simulink model "VDSE_2018a"  (R2018a)
settings: Solver=ode5  StartTime=0.0  StopTime=T_simulation  FixedStep=simulation_step_time  RelTol=1e-3
values from neighbouring files (symbols this model uses):
  A = 2    [vehicle_parameters_script.m]
  bump_height = 0    [vehicle_parameters_script.m]
  bump_length = 1    [vehicle_parameters_script.m]
  bump_time = 1    [vehicle_parameters_script.m]
  Bxf = 17.156    [BCD_Parameters.m]
  Bxr = 17.156    [BCD_Parameters.m]
  Byf = 12.71    [BCD_Parameters.m]
  Byr = 12.71    [BCD_Parameters.m]
  cd = 0.35    [vehicle_parameters_script.m]
  central_diff = 1    [vehicle_parameters_script.m]
  cF = 5000    [vehicle_parameters_script.m]
  clF = -0.15    [vehicle_parameters_script.m]
  clR = -0.20    (= -0.2)    [vehicle_parameters_script.m]
  cp_FA = 30    [vehicle_parameters_script.m]
  cp_RA = 13    [vehicle_parameters_script.m]
  cR = 5000    [vehicle_parameters_script.m]
  ctF = tireF.VERTICAL_DAMPING    [vehicle_parameters_script.m]
  ctR = tireR.VERTICAL_DAMPING    [vehicle_parameters_script.m]
  Cxf = 1.406    [BCD_Parameters.m]
  Cxr = 1.406    [BCD_Parameters.m]
  Cyf = 1.63    [BCD_Parameters.m]
  Cyr = 1.63    [BCD_Parameters.m]
  Dxf = 1.2    [BCD_Parameters.m]
  Dxr = 1.2    [BCD_Parameters.m]
  Dyf = 1.1    [BCD_Parameters.m]
  Dyr = 1.8    [BCD_Parameters.m]
  enableDriverControl = 0    [vehicle_parameters_script.m]
  enableLongDynamics = 1    [vehicle_parameters_script.m]
  enablePowertrain = 1    [vehicle_parameters_script.m]
  front_dr = 3.8    [vehicle_parameters_script.m]
  g = 9.806    [vehicle_parameters_script.m]
  Gear_numbers = [1 2 3 4 5 6]    [vehicle_parameters_script.m]
  GR = [2.9 1.8 1.3 1 0.85 0.75]    [vehicle_parameters_script.m]
  hcog = 0.5    [vehicle_parameters_script.m]
  hpc = 0.0    (= 0)    [vehicle_parameters_script.m]
  hrcF = 0.3    [vehicle_parameters_script.m]
  hrcg = (hrcF*lR+hrcR*lF)/(lF+lR)    (= 0.25108)    [vehicle_parameters_script.m]
  hrcR = 0.2    [vehicle_parameters_script.m]
  huFcog = 0.32    [vehicle_parameters_script.m]
  huRcog = 0.32    [vehicle_parameters_script.m]
  initial_gear = 1    [vehicle_parameters_script.m]
  JwF = 2.45    [vehicle_parameters_script.m]
  JwR = 2.45    [vehicle_parameters_script.m]
  Jx = 430    [vehicle_parameters_script.m]
  Jy = 1309    [vehicle_parameters_script.m]
  Jz = 1461    [vehicle_parameters_script.m]
  kF = 40000    [vehicle_parameters_script.m]
  kR = 35000    [vehicle_parameters_script.m]
  kRF = 0    [vehicle_parameters_script.m]
  kRR = 0    [vehicle_parameters_script.m]
  ktF = tireF.VERTICAL_STIFFNESS    [vehicle_parameters_script.m]
  ktR = tireR.VERTICAL_STIFFNESS    [vehicle_parameters_script.m]
  lF = 1.223    [vehicle_parameters_script.m]
  lR = l-lF    (= 1.277)    [vehicle_parameters_script.m]
  m = 1310    [vehicle_parameters_script.m]
  max_pressure = 1000    [vehicle_parameters_script.m]
  maxrpm = 4000    [vehicle_parameters_script.m]
  mF = 45    [vehicle_parameters_script.m]
  minrpm = 1500    [vehicle_parameters_script.m]
  mR = 50    [vehicle_parameters_script.m]
  output_samping_time = 0.001    [vehicle_parameters_script.m]
  phi0 = 0    [vehicle_parameters_script.m]
  phi_dot0 = 0    [vehicle_parameters_script.m]
  psi0 = 0    [vehicle_parameters_script.m]
  psi_dot0 = 0    [vehicle_parameters_script.m]
  rear_dr = 3.8    [vehicle_parameters_script.m]
  requested_speed = 100/3.6    (= 27.7777777778)    [vehicle_parameters_script.m]
  rF = tireF.UNLOADED_RADIUS    [vehicle_parameters_script.m]
  rho = 1.2    [vehicle_parameters_script.m]
  RPMME = Engine(:,1)    [vehicle_parameters_script.m]
  rR = tireR.UNLOADED_RADIUS    [vehicle_parameters_script.m]
  steer_ratio = 13.25    [vehicle_parameters_script.m]
  TFL = 0    [vehicle_parameters_script.m]
  TFR = 0    [vehicle_parameters_script.m]
  theta0 = 0    [vehicle_parameters_script.m]
  theta_dot0 = 0    [vehicle_parameters_script.m]
  TorqueME = []    [vehicle_parameters_script.m]
  TRL = 0    [vehicle_parameters_script.m]
  TRR = 0    [vehicle_parameters_script.m]
  Vx0 = 100/3.6    (= 27.7777777778)    [vehicle_parameters_script.m]
  Vy0 = 0    [vehicle_parameters_script.m]
  Vz0 = 0    [vehicle_parameters_script.m]
  wF = 1.578    [vehicle_parameters_script.m]
  wR = 1.544    [vehicle_parameters_script.m]
  x0 = 0    [vehicle_parameters_script.m]
  xcog_overall = (2*mR*xR+2*xF*mF+m*xs)/(m+2*mF+2*mR)    (= 1.23475333333)    [vehicle_parameters_script.m]
  y0 = 0    [vehicle_parameters_script.m]
  z0 = 0    [vehicle_parameters_script.m]
  zFL0 = 0    [vehicle_parameters_script.m]
  zFL_dot0 = 0    [vehicle_parameters_script.m]
  zFR0 = 0    [vehicle_parameters_script.m]
  zFR_dot0 = 0    [vehicle_parameters_script.m]
  zRL0 = 0    [vehicle_parameters_script.m]
  zRL_dot0 = 0    [vehicle_parameters_script.m]
  zRR0 = 0    [vehicle_parameters_script.m]
  zRR_dot0 = 0    [vehicle_parameters_script.m]
undefined symbols (not defined in the file or in its folder): exf, exr, eyf, eyr, FNOMINf, FNOMINr, PCX1f, PCX1r, PCY1f, PCY1r, PDX1f, PDX1r, PDX2f, PDX2r, PDY1f, PDY1r, PDY2f, PDY2r, PDY3f, PDY3r, PEX1f, PEX1r, PEX2f, PEX2r, PEX3f, PEX3r, PEX4f, PEX4r, PEY1f, PEY1r, PEY2f, PEY2r, PEY3f, PEY3r, PEY4f, PEY4r, PHX1f, PHX1r, PHX2f, PHX2r, PHY1f, PHY1r, PHY2f, PHY2r, PHY3f, PHY3r, PKX1f, PKX1r, PKX2f, PKX2r, PKX3f, PKX3r, PKY1f, PKY1r, PKY2f, PKY2r, PKY3f, PKY3r, PVX1f, PVX1r ... (+122)
libraries: simulink x7, mfeval_LIB x4
(part 3 of 6)

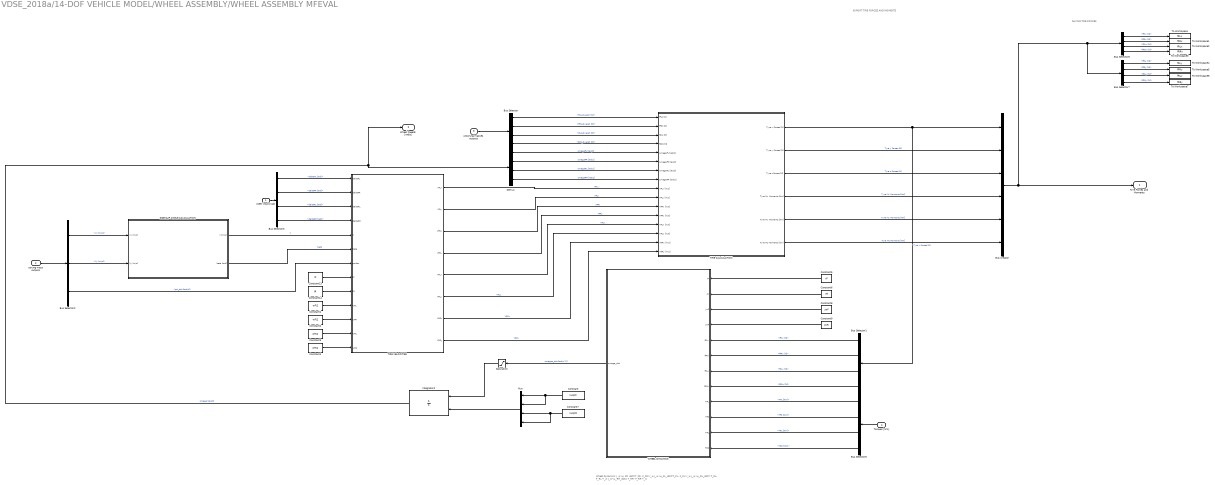
== system VDSE_2018a/14-DOF VEHICLE MODEL/WHEEL ASSEMBLY/WHEEL ASSEMBLY MFEVAL ==
  note: EXPORT TIRE FORCES AND MOMENTS
  note: Wheel Dynamics:
      |
      | J_w∙ω_FR_dot=T_FR- F_FR∙r_w
      | J_w∙ω_FL_dot=T_FL- F_FL∙r_w
      | J_w∙ω_RL_dot= T_RL- F_RL∙r_w
      | J_w∙ω_RR_dot= T_RR- F_RR∙r_w
  note: SAVING TIRE FORCES
  steer input [rad] : Inport
  sprung mass outputs : Inport  Port=2
  unsprung masses outputs : Inport  Port=3
  Torques [Nm] : Inport  Port=4
  Bus Creator : BusCreator  Inputs=6
  Bus Selector : BusSelector  OutputSignals=Unsprung masses z Forces [N].FLz_Overall [N],Unsprung masses z Forces [N].FRz_Overall [N],Unsprung masses z Forces [N].RLz_Overall [N],Unsprung masses z Forces [N].RRz_Overall [N]
  Bus Selector1 : BusSelector  OutputSignals=fFLx [N],fFRx [N],fRLx [N],fRRx [N]
  Bus Selector2 : BusSelector  OutputSignals=Longitudinal Dynamics.Vx [m/s],Lateral Dynamics.Vy [m/s],Yaw dynamics.psi_dot [rad/s]
  Bus Selector3 : BusSelector  OutputSignals=Steering.deltaFL [rad],Steering.deltaFR [rad],Steering.deltaRL [rad],Steering.deltaRR [rad]
  Bus Selector5 : BusSelector  OutputSignals=TFL [Nm],TFR [Nm],TRL [Nm],TRR [Nm]
  Bus Selector6 : BusSelector  OutputSignals=Tyre x Forces [N].fFLx [N],Tyre x Forces [N].fFRx [N],Tyre x Forces [N].fRLx [N],Tyre x Forces [N].fRRx [N]
  Bus Selector7 : BusSelector  OutputSignals=Tyre y Forces [N].fFLy [N],Tyre y Forces [N].fFRy [N],Tyre y Forces [N].fRLy [N],Tyre y Forces [N].fRRy [N]
  Constant : Constant  Value=Vx0/rF
  Constant1 : Constant  Value=wF/2
  Constant13 : Constant  Value=lF
  Constant14 : Constant  Value=lR
  Constant2 : Constant  Value=wF/2
  Constant3 : Constant  Value=wR/2
  Constant4 : Constant  Value=wR/2
  Constant5 : Constant  Value=rF
  Constant6 : Constant  Value=rR
  Constant7 : Constant  Value=Vx0/rR
  Constant8 : Constant  Value=JwF
  Constant9 : Constant  Value=JwR
  Demux : Demux
  Integrator2 : Integrator  InitialConditionSource=external
  Mux : Mux
  SIDE SLIP ANGLE CALCULATION : Subsystem
  Saturation : Saturate  UpperLimit=5000  LowerLimit=-5000
  TIRE CALCULATION : Subsystem
  TIRE VELOCITIES : MATLAB Function  TreatAsAtomicUnit=on
  To Workspace : ToWorkspace  VariableName=fFLx  SaveFormat=Timeseries  SampleTime=-1
  To Workspace1 : ToWorkspace  VariableName=fFRx  SaveFormat=Timeseries  SampleTime=-1
  To Workspace2 : ToWorkspace  VariableName=fRLx  SaveFormat=Timeseries  SampleTime=-1
  To Workspace3 : ToWorkspace  VariableName=fRRx  SaveFormat=Timeseries  SampleTime=-1
  To Workspace4 : ToWorkspace  VariableName=fFLy  SaveFormat=Timeseries  SampleTime=-1
  To Workspace5 : ToWorkspace  VariableName=fFRy  SaveFormat=Timeseries  SampleTime=-1
  To Workspace6 : ToWorkspace  VariableName=fRLy  SaveFormat=Timeseries  SampleTime=-1
  To Workspace7 : ToWorkspace  VariableName=fRRy  SaveFormat=Timeseries  SampleTime=-1
  WHEEL DYNAMICS : MATLAB Function  TreatAsAtomicUnit=on
  Tyre Forces and Moments : Outport
  Wheel Speeds [rad/s] : Outport  Port=2
  wires:
  TIRE CALCULATION/4(Tyre Mx Moments [Nm]) -> Bus Creator/4  "Tyre Mx Moments [Nm]"
  Bus Selector7/4 -> To Workspace7/1  "<fRRy [N]>"
  Bus Selector7/3 -> To Workspace6/1  "<fRLy [N]>"
  Bus Selector7/2 -> To Workspace5/1  "<fFRy [N]>"
  Bus Selector7/1 -> To Workspace4/1  "<fFLy [N]>"
  Bus Selector6/4 -> To Workspace3/1  "<fRRx [N]>"
  Bus Selector6/3 -> To Workspace2/1  "<fRLx [N]>"
  Bus Selector6/2 -> To Workspace1/1  "<fFRx [N]>"
  Bus Selector6/1 -> To Workspace/1  "<fFLx [N]>"
  Torques [Nm]/1 -> Bus Selector5/1
  Bus Creator/1 -> Bus Selector6/1, Bus Selector7/1, Tyre Forces and Moments/1
  steer input [rad]/1 -> Bus Selector3/1
  Bus Selector3/3 -> TIRE VELOCITIES/3(deltaRL)  "<deltaRL [rad]>"
  Bus Selector3/1 -> TIRE VELOCITIES/1(deltaFL)  "<deltaFL [rad]>"
  Bus Selector3/4 -> TIRE VELOCITIES/4(deltaRR)  "<deltaRR [rad]>"
  Bus Selector3/2 -> TIRE VELOCITIES/2(deltaFR)  "<deltaFR [rad]>"
  sprung mass outputs/1 -> Bus Selector2/1
  Bus Selector2/3 -> TIRE VELOCITIES/7(psidot)  "<psi_dot [rad/s]>"
  unsprung masses outputs/1 -> Bus Selector/1
  Bus Selector/2 -> TIRE CALCULATION/2(fFRz [N])  "<FRz_Overall [N]>"
  Bus Selector/3 -> TIRE CALCULATION/3(fRLz [N])  "<RLz_Overall [N]>"
  Bus Selector/4 -> TIRE CALCULATION/4(fRRz [N])  "<RRz_Overall [N]>"
  Bus Selector/1 -> TIRE CALCULATION/1(fFLz [N])  "<FLz_Overall [N]>"
  SIDE SLIP ANGLE CALCULATION/1(V [m/s]) -> TIRE VELOCITIES/5(V)  "V"
  SIDE SLIP ANGLE CALCULATION/2(beta [rad]) -> TIRE VELOCITIES/6(beta)  "beta"
  TIRE VELOCITIES/8(VRRy) -> TIRE CALCULATION/16(VRRy [m/s])  "VRRy"
  TIRE VELOCITIES/7(VRRx) -> TIRE CALCULATION/15(VRRx [m/s])  "VRRx"
  TIRE VELOCITIES/6(VRLy) -> TIRE CALCULATION/14(VRLy [m/s])  "VRLy"
  TIRE VELOCITIES/3(VFRx) -> TIRE CALCULATION/11(VFRx [m/s])  "VFRx"
  Bus Selector1/1 -> WHEEL DYNAMICS/5(fFLx)  "<fFLx [N]>"
  Constant9/1 -> WHEEL DYNAMICS/4(JwR)
  Constant3/1 -> TIRE VELOCITIES/12(wRL)
  TIRE VELOCITIES/5(VRLx) -> TIRE CALCULATION/13(VRLx [m/s])  "VRLx"
  Constant2/1 -> TIRE VELOCITIES/11(wFR)
  Demux/4 -> TIRE CALCULATION/8(omegaRR [rad/s])  "omegaRR [rad/s]"
  Constant/1 -> Mux/1, Mux/2
  Demux/3 -> TIRE CALCULATION/7(omegaRL [rad/s])  "omegaRL [rad/s]"
  Demux/1 -> TIRE CALCULATION/5(omegaFL [rad/s])  "omegaFL [rad/s]"
  WHEEL DYNAMICS/1(omega_dot) -> Saturation/1  "omegas_dot [rad/s^2]"
  Constant14/1 -> TIRE VELOCITIES/9(lR)
  Constant8/1 -> WHEEL DYNAMICS/3(JwF)
  Constant1/1 -> TIRE VELOCITIES/10(wFL)
  Mux/1 -> Integrator2/2
  Constant5/1 -> WHEEL DYNAMICS/1(rF)
  Constant13/1 -> TIRE VELOCITIES/8(lF)
  Integrator2/1 -> Wheel Speeds [rad/s]/1, Demux/1  "omega [rad/s]"
  Bus Selector1/2 -> WHEEL DYNAMICS/6(fFRx)  "<fFRx [N]>"
  Constant4/1 -> TIRE VELOCITIES/13(wRR)
  Bus Selector1/3 -> WHEEL DYNAMICS/7(fRLx)  "<fRLx [N]>"
  TIRE VELOCITIES/4(VFRy) -> TIRE CALCULATION/12(VFRy [m/s])  "VFRy"
  TIRE VELOCITIES/1(VFLx) -> TIRE CALCULATION/9(VFLx [m/s])  "VFLx"
  Constant6/1 -> WHEEL DYNAMICS/2(rR)
  Demux/2 -> TIRE CALCULATION/6(omegaFR [rad/s])  "omegaFR [rad/s]"
  Constant7/1 -> Mux/4, Mux/3
  Bus Selector1/4 -> WHEEL DYNAMICS/8(fRRx)  "<fRRx [N]>"
  TIRE VELOCITIES/2(VFLy) -> TIRE CALCULATION/10(VFLy [m/s])  "VFLy"
  TIRE CALCULATION/1(Tyre x Forces [N]) -> Bus Creator/1, Bus Selector1/1  "Tyre x Forces [N]"
  TIRE CALCULATION/2(Tyre y Forces [N]) -> Bus Creator/2  "Tyre y Forces [N]"
  TIRE CALCULATION/6(Tyre Mz Moments [Nm]) -> Bus Creator/6  "Tyre Mz Moments [Nm]"
  TIRE CALCULATION/3(Tyre z Forces [N]) -> Bus Creator/3  "Tyre z Forces [N]"
  TIRE CALCULATION/5(Tyre My Moments [Nm]) -> Bus Creator/5  "Tyre My Moments [Nm]"
  Bus Selector2/2 -> SIDE SLIP ANGLE CALCULATION/2(Vy [m/s])  "<Vy [m/s]>"
  Bus Selector2/1 -> SIDE SLIP ANGLE CALCULATION/1(Vx [m/s])  "<Vx [m/s]>"
  Bus Selector5/1 -> WHEEL DYNAMICS/9(TFL)  "<TFL [Nm]>"
  Bus Selector5/2 -> WHEEL DYNAMICS/10(TFR)  "<TFR [Nm]>"
  Bus Selector5/3 -> WHEEL DYNAMICS/11(TRL)  "<TRL [Nm]>"
  Bus Selector5/4 -> WHEEL DYNAMICS/12(TRR)  "<TRR [Nm]>"
  Saturation/1 -> Integrator2/1

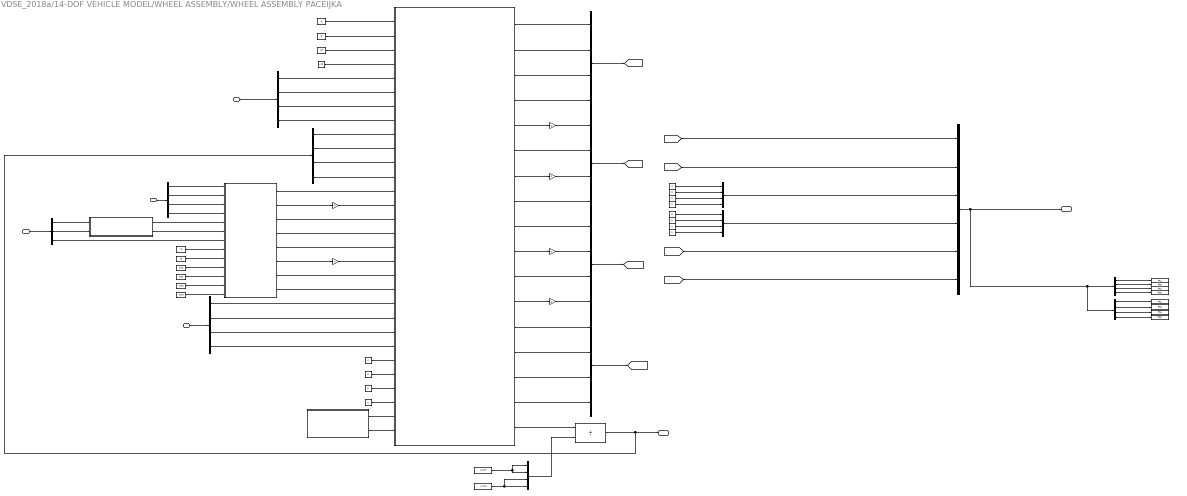
== system VDSE_2018a/14-DOF VEHICLE MODEL/WHEEL ASSEMBLY/WHEEL ASSEMBLY PACEIJKA ==
  note: EXPORTING TIRE FORCES AND MOMENTS
  note: SAVING TIRE FORCES
  steer input [rad] : Inport
  sprung mass outputs : Inport  Port=2
  unsprung masses outputs : Inport  Port=3
  Torques [Nm] : Inport  Port=4
  Bus Creator : BusCreator  Inputs=6
  Bus Creator{1..4,7..8} (6 alike) : BusCreator  Inputs=4
  Bus Selector : BusSelector  OutputSignals=Unsprung masses z Forces [N].FLz_Overall [N],Unsprung masses z Forces [N].FRz_Overall [N],Unsprung masses z Forces [N].RLz_Overall [N],Unsprung masses z Forces [N].RRz_Overall [N]
  Bus Selector2 : BusSelector  OutputSignals=Longitudinal Dynamics.Vx [m/s],Lateral Dynamics.Vy [m/s],Yaw dynamics.psi_dot [rad/s]
  Bus Selector3 : BusSelector  OutputSignals=Steering.deltaFL [rad],Steering.deltaFR [rad],Steering.deltaRL [rad],Steering.deltaRR [rad]
  Bus Selector5 : BusSelector  OutputSignals=TFL [Nm],TFR [Nm],TRL [Nm],TRR [Nm]
  Bus Selector6 : BusSelector  OutputSignals=Tyre x Forces [N].fFLx [N],Tyre x Forces [N].fFRx [N],Tyre x Forces [N].fRLx [N],Tyre x Forces [N].fRRx [N]
  Bus Selector7 : BusSelector  OutputSignals=Tyre y Forces [N].fFLy [N],Tyre y Forces [N].fFRy [N],Tyre y Forces [N].fRLy [N],Tyre y Forces [N].fRRy [N]
  Constant{,26..28} (4 alike) : Constant  Value=0
  Constant1 : Constant  Value=wF/2
  Constant13 : Constant  Value=lF
  Constant14 : Constant  Value=lR
  Constant2 : Constant  Value=wF/2
  Constant20 : Constant  Value=rF
  Constant21 : Constant  Value=rR
  Constant22 : Constant  Value=JwF
  Constant23 : Constant  Value=JwR
  Constant24 : Constant  Value=Vx0/rF
  Constant25 : Constant  Value=Vx0/rR
  Constant3 : Constant  Value=wR/2
  Constant4 : Constant  Value=wR/2
  Demux1 : Demux
  Gain{,1..5} (6 alike) : Gain  Gain=-1
  Integrator1 : Integrator  InitialConditionSource=external
  Mux2 : Mux
  SIDE SLIP ANGLE CALCULATION : Subsystem
  TIRE FORCES AND WHEEL DYNAMICS : MATLAB Function  TreatAsAtomicUnit=on
  TIRE PARAMETERS : Subsystem
  TIRE VELOCITIES : MATLAB Function  TreatAsAtomicUnit=on
  To Workspace : ToWorkspace  VariableName=fFLx  SaveFormat=Timeseries  SampleTime=-1
  To Workspace1 : ToWorkspace  VariableName=fFRx  SaveFormat=Timeseries  SampleTime=-1
  To Workspace2 : ToWorkspace  VariableName=fRLx  SaveFormat=Timeseries  SampleTime=-1
  To Workspace3 : ToWorkspace  VariableName=fRRx  SaveFormat=Timeseries  SampleTime=-1
  To Workspace4 : ToWorkspace  VariableName=fFLy  SaveFormat=Timeseries  SampleTime=-1
  To Workspace5 : ToWorkspace  VariableName=fFRy  SaveFormat=Timeseries  SampleTime=-1
  To Workspace6 : ToWorkspace  VariableName=fRLy  SaveFormat=Timeseries  SampleTime=-1
  To Workspace7 : ToWorkspace  VariableName=fRRy  SaveFormat=Timeseries  SampleTime=-1
  Zero{,1..7} (8 alike) : Constant  Value=0  OutDataTypeStr=Inherit: Inherit via back propagation
  Tyre Forces and Moments : Outport
  Wheel Speeds [rad/s] : Outport  Port=2
  wires:
  Zero/1 -> Bus Creator3/1  "fFLz [N]"
  Zero2/1 -> Bus Creator3/3  "fRLz [N]"
  Zero4/1 -> Bus Creator4/1  "mFLx [Nm]"
  Zero1/1 -> Bus Creator3/2  "fFRz [N]"
  Zero7/1 -> Bus Creator4/4  "mRRx [Nm]"
  Zero5/1 -> Bus Creator4/2  "mFRx [Nm]"
  Zero3/1 -> Bus Creator3/4  "fRRz [N]"
  Zero6/1 -> Bus Creator4/3  "mRLx [Nm]"
  Bus Creator2/1 -> [Tyre_y_Forces]  "Tyre y Forces [N]"
  TIRE FORCES AND WHEEL DYNAMICS/7(fRLy) -> Gain2/1  "fRLy [N]"
  TIRE FORCES AND WHEEL DYNAMICS/5(fFLy) -> Gain3/1  "fFLy [N]"
  Bus Creator1/1 -> [Tyre_x_Forces]  "Tyre x Forces [N]"
  TIRE VELOCITIES/8(VRRy) -> TIRE FORCES AND WHEEL DYNAMICS/20(VRRy)  "VRRy"
  TIRE VELOCITIES/7(VRRx) -> TIRE FORCES AND WHEEL DYNAMICS/19(VRRx)  "VRRx"
  Integrator1/1 -> Wheel Speeds [rad/s]/1, Demux1/1  "omega [rad/s]"
  Demux1/4 -> TIRE FORCES AND WHEEL DYNAMICS/12(omegaRR)
  Demux1/3 -> TIRE FORCES AND WHEEL DYNAMICS/11(omegaRL)
  Demux1/2 -> TIRE FORCES AND WHEEL DYNAMICS/10(omegaFR)
  Demux1/1 -> TIRE FORCES AND WHEEL DYNAMICS/9(omegaFL)
  TIRE FORCES AND WHEEL DYNAMICS/17(omega_dot) -> Integrator1/1  "omegas_dot [rad/s^2]"
  Constant25/1 -> Mux2/4, Mux2/3
  Mux2/1 -> Integrator1/2
  Constant24/1 -> Mux2/1, Mux2/2
  Constant21/1 -> TIRE FORCES AND WHEEL DYNAMICS/2(rR)
  Constant23/1 -> TIRE FORCES AND WHEEL DYNAMICS/4(JwR)
  Constant22/1 -> TIRE FORCES AND WHEEL DYNAMICS/3(JwF)
  Constant20/1 -> TIRE FORCES AND WHEEL DYNAMICS/1(rF)
  TIRE VELOCITIES/2(VFLy) -> Gain/1  "VFLy"
  TIRE VELOCITIES/1(VFLx) -> TIRE FORCES AND WHEEL DYNAMICS/13(VFLx)  "VFLx"
  TIRE VELOCITIES/4(VFRy) -> TIRE FORCES AND WHEEL DYNAMICS/16(VFRy)  "VFRy"
  Constant4/1 -> TIRE VELOCITIES/13(wRR)
  Constant13/1 -> TIRE VELOCITIES/8(lF)
  Constant1/1 -> TIRE VELOCITIES/10(wFL)
  Constant14/1 -> TIRE VELOCITIES/9(lR)
  Constant2/1 -> TIRE VELOCITIES/11(wFR)
  TIRE VELOCITIES/5(VRLx) -> TIRE FORCES AND WHEEL DYNAMICS/17(VRLx)  "VRLx"
  Constant3/1 -> TIRE VELOCITIES/12(wRL)
  TIRE VELOCITIES/3(VFRx) -> TIRE FORCES AND WHEEL DYNAMICS/15(VFRx)  "VFRx"
  TIRE VELOCITIES/6(VRLy) -> Gain1/1  "VRLy"
  SIDE SLIP ANGLE CALCULATION/2(beta [rad]) -> TIRE VELOCITIES/6(beta)  "beta"
  SIDE SLIP ANGLE CALCULATION/1(V [m/s]) -> TIRE VELOCITIES/5(V)  "V"
  Bus Selector/1 -> TIRE FORCES AND WHEEL DYNAMICS/5(fFLz)  "<FLz_Overall [N]>"
  Bus Selector/4 -> TIRE FORCES AND WHEEL DYNAMICS/8(fRRz)  "<RRz_Overall [N]>"
  Bus Selector/3 -> TIRE FORCES AND WHEEL DYNAMICS/7(fRLz)  "<RLz_Overall [N]>"
  Bus Selector/2 -> TIRE FORCES AND WHEEL DYNAMICS/6(fFRz)  "<FRz_Overall [N]>"
  unsprung masses outputs/1 -> Bus Selector/1
  sprung mass outputs/1 -> Bus Selector2/1
  Bus Selector3/2 -> TIRE VELOCITIES/2(deltaFR)  "<deltaFR [rad]>"
  Bus Selector3/4 -> TIRE VELOCITIES/4(deltaRR)  "<deltaRR [rad]>"
  Bus Selector3/1 -> TIRE VELOCITIES/1(deltaFL)  "<deltaFL [rad]>"
  Bus Selector3/3 -> TIRE VELOCITIES/3(deltaRL)  "<deltaRL [rad]>"
  steer input [rad]/1 -> Bus Selector3/1
  Bus Creator/1 -> Bus Selector7/1, Bus Selector6/1, Tyre Forces and Moments/1
  Torques [Nm]/1 -> Bus Selector5/1
  Bus Selector6/1 -> To Workspace/1  "<fFLx [N]>"
  Bus Selector6/2 -> To Workspace1/1  "<fFRx [N]>"
  Bus Selector6/3 -> To Workspace2/1  "<fRLx [N]>"
  Bus Selector6/4 -> To Workspace3/1  "<fRRx [N]>"
  Bus Selector7/1 -> To Workspace4/1  "<fFLy [N]>"
  Bus Selector7/2 -> To Workspace5/1  "<fFRy [N]>"
  Bus Selector7/3 -> To Workspace6/1  "<fRLy [N]>"
  Bus Selector7/4 -> To Workspace7/1  "<fRRy [N]>"
  [Tyre_y_Moments] -> Bus Creator/5  "Tyre My Moments [Nm]"
  Constant/1 -> TIRE FORCES AND WHEEL DYNAMICS/25(gammaFL)
  Constant26/1 -> TIRE FORCES AND WHEEL DYNAMICS/26(gammaFR)
  Constant27/1 -> TIRE FORCES AND WHEEL DYNAMICS/27(gammaRL)
  Constant28/1 -> TIRE FORCES AND WHEEL DYNAMICS/28(gammaRR)
  TIRE PARAMETERS/1(Tire Parameters Front Axle) -> TIRE FORCES AND WHEEL DYNAMICS/29(TireParams_front)
  TIRE PARAMETERS/2(Tire Parameters Rear Axle) -> TIRE FORCES AND WHEEL DYNAMICS/30(TireParams_rear)
  Gain/1 -> TIRE FORCES AND WHEEL DYNAMICS/14(VFLy)  "VFLy"
  Gain1/1 -> TIRE FORCES AND WHEEL DYNAMICS/18(VRLy)  "VRLy"
  TIRE FORCES AND WHEEL DYNAMICS/1(fFLx) -> Bus Creator1/1  "fFLx [N]"
  TIRE FORCES AND WHEEL DYNAMICS/2(fFRx) -> Bus Creator1/2  "fFRx [N]"
  TIRE FORCES AND WHEEL DYNAMICS/3(fRLx) -> Bus Creator1/3  "fRLx [N]"
  TIRE FORCES AND WHEEL DYNAMICS/4(fRRx) -> Bus Creator1/4  "fRRx [N]"
  Gain3/1 -> Bus Creator2/1  "fFLy [N]"
  TIRE FORCES AND WHEEL DYNAMICS/6(fFRy) -> Bus Creator2/2  "fFRy [N]"
  Gain2/1 -> Bus Creator2/3  "fRLy [N]"
  TIRE FORCES AND WHEEL DYNAMICS/8(fRRy) -> Bus Creator2/4  "fRRy [N]"
  [Tyre_x_Forces] -> Bus Creator/1  "Tyre x Forces [N]"
  [Tyre_y_Forces] -> Bus Creator/2  "Tyre y Forces [N]"
  Bus Creator3/1 -> Bus Creator/3  "Tyre z Forces [N]"
  Bus Creator4/1 -> Bus Creator/4  "Tyre Mx Moments [Nm]"
  [Tyre_z_Moments] -> Bus Creator/6  "Tyre Mz Moments [Nm]"
  TIRE FORCES AND WHEEL DYNAMICS/9(mFLz) -> Bus Creator7/1  "mFLz [Nm]"
  TIRE FORCES AND WHEEL DYNAMICS/10(mFRz) -> Gain4/1  "mFRz [Nm]"
  Gain4/1 -> Bus Creator7/2  "mFRz [Nm]"
  TIRE FORCES AND WHEEL DYNAMICS/11(mRLz) -> Bus Creator7/3  "mRLz [Nm]"
  TIRE FORCES AND WHEEL DYNAMICS/12(mRRz) -> Gain5/1  "mRRz [Nm]"
  Gain5/1 -> Bus Creator7/4  "mRRz [Nm]"
  TIRE FORCES AND WHEEL DYNAMICS/13(mFLy) -> Bus Creator8/1  "mFLy [Nm]"
  TIRE FORCES AND WHEEL DYNAMICS/14(mFRy) -> Bus Creator8/2  "mFRy [Nm]"
  TIRE FORCES AND WHEEL DYNAMICS/15(mRLy) -> Bus Creator8/3  "mRLy [Nm]"
  TIRE FORCES AND WHEEL DYNAMICS/16(mRRy) -> Bus Creator8/4  "mRRy [Nm]"
  Bus Creator7/1 -> [Tyre_z_Moments]  "Tyre Mz Moments [Nm]"
  Bus Creator8/1 -> [Tyre_y_Moments]  "Tyre My Moments [Nm]"
  Bus Selector2/1 -> SIDE SLIP ANGLE CALCULATION/1(Vx [m/s])  "<Vx [m/s]>"
  Bus Selector2/2 -> SIDE SLIP ANGLE CALCULATION/2(Vy [m/s])  "<Vy [m/s]>"
  Bus Selector2/3 -> TIRE VELOCITIES/7(psidot)  "<psi_dot [rad/s]>"
  Bus Selector5/1 -> TIRE FORCES AND WHEEL DYNAMICS/21(TFL)  "<TFL [Nm]>"
  Bus Selector5/2 -> TIRE FORCES AND WHEEL DYNAMICS/22(TFR)  "<TFR [Nm]>"
  Bus Selector5/3 -> TIRE FORCES AND WHEEL DYNAMICS/23(TRL)  "<TRL [Nm]>"
  Bus Selector5/4 -> TIRE FORCES AND WHEEL DYNAMICS/24(TRR)  "<TRR [Nm]>"

== system VDSE_2018a/14-DOF VEHICLE MODEL/EQUATIONS OF MOTION FOR CHASSIS/Pitch Dynamics/Downforce ==
  Vx : Inport
  Gain : Gain  Gain=-0.5*rho*clF*A
  Gain{1,3,5,7} (4 alike) : Gain  Gain=0.5
  Gain2 : Gain  Gain=-0.5*rho*clF*A
  Gain4 : Gain  Gain=-0.5*rho*clR*A
  Gain6 : Gain  Gain=-0.5*rho*clR*A
  Square{,1..3} (4 alike) : Math  Operator=square  SaturateOnIntegerOverflow=on
  fFLz_overall : Outport
  fFRz_overall : Outport  Port=2
  fRLz_overall : Outport  Port=3
  fRRz_overall : Outport  Port=4
  wires:
  Gain/1 -> Gain1/1
  Square/1 -> Gain/1
  Gain1/1 -> fFLz_overall/1
  Square1/1 -> Gain2/1
  Gain2/1 -> Gain3/1
  Gain3/1 -> fFRz_overall/1
  Vx/1 -> Square/1, Square1/1, Square2/1, Square3/1
  Gain6/1 -> Gain7/1
  Square3/1 -> Gain6/1
  Square2/1 -> Gain4/1
  Gain4/1 -> Gain5/1
  Gain5/1 -> fRLz_overall/1
  Gain7/1 -> fRRz_overall/1

== system VDSE_2018a/14-DOF VEHICLE MODEL/EQUATIONS OF MOTION FOR CHASSIS/Roll Dynamics/Downforce ==
  Vx : Inport
  Gain : Gain  Gain=-0.5*rho*clF*A
  Gain{1,3,5,7} (4 alike) : Gain  Gain=0.5
  Gain2 : Gain  Gain=-0.5*rho*clF*A
  Gain4 : Gain  Gain=-0.5*rho*clR*A
  Gain6 : Gain  Gain=-0.5*rho*clR*A
  Square{,1..3} (4 alike) : Math  Operator=square  SaturateOnIntegerOverflow=on
  fFLz_overall : Outport
  fFRz_overall : Outport  Port=2
  fRLz_overall : Outport  Port=3
  fRRz_overall : Outport  Port=4
  wires:
  Gain/1 -> Gain1/1
  Square/1 -> Gain/1
  Gain1/1 -> fFLz_overall/1
  Square1/1 -> Gain2/1
  Gain2/1 -> Gain3/1
  Gain3/1 -> fFRz_overall/1
  Vx/1 -> Square/1, Square1/1, Square2/1, Square3/1
  Gain6/1 -> Gain7/1
  Square3/1 -> Gain6/1
  Square2/1 -> Gain4/1
  Gain4/1 -> Gain5/1
  Gain5/1 -> fRLz_overall/1
  Gain7/1 -> fRRz_overall/1

== system VDSE_2018a/14-DOF VEHICLE MODEL/EQUATIONS OF MOTION FOR CHASSIS/Vertical Dynamics/Downforce ==
  Vx : Inport
  Gain : Gain  Gain=-0.5*rho*clF*A
  Gain{1,3,5,7} (4 alike) : Gain  Gain=0.5
  Gain2 : Gain  Gain=-0.5*rho*clF*A
  Gain4 : Gain  Gain=-0.5*rho*clR*A
  Gain6 : Gain  Gain=-0.5*rho*clR*A
  Square{,1..3} (4 alike) : Math  Operator=square  SaturateOnIntegerOverflow=on
  fFLz_overall : Outport
  fFRz_overall : Outport  Port=2
  fRLz_overall : Outport  Port=3
  fRRz_overall : Outport  Port=4
  wires:
  Gain/1 -> Gain1/1
  Square/1 -> Gain/1
  Gain1/1 -> fFLz_overall/1
  Square1/1 -> Gain2/1
  Gain2/1 -> Gain3/1
  Gain3/1 -> fFRz_overall/1
  Vx/1 -> Square/1, Square1/1, Square2/1, Square3/1
  Gain6/1 -> Gain7/1
  Square3/1 -> Gain6/1
  Square2/1 -> Gain4/1
  Gain4/1 -> Gain5/1
  Gain5/1 -> fRLz_overall/1
  Gain7/1 -> fRRz_overall/1

== system VDSE_2018a/14-DOF VEHICLE MODEL/POWERTRAIN AND BRAKES/Engine and Gear Box/Subsystem ==
  Gear_Ratio : Inport
  Front shaft rotational velocity [rpm] : Inport  Port=2
  Rear shaft rotational velocity [rpm] : Inport  Port=3
  Add : Sum
  Gain15 : Gain  Gain=1-central_diff
  Gain16 : Gain  Gain=central_diff
  Product2 : Product
  Product3 : Product
  Engine shaft rotational velocity [rpm] : Outport
  wires:
  Front shaft rotational velocity [rpm]/1 -> Product2/2
  Gear_Ratio/1 -> Product3/1, Product2/1
  Product3/1 -> Gain15/1  "rpm"
  Product2/1 -> Gain16/1
  Gain15/1 -> Add/2
  Rear shaft rotational velocity [rpm]/1 -> Product3/2
  Gain16/1 -> Add/1
  Add/1 -> Engine shaft rotational velocity [rpm]/1

== system VDSE_2018a/14-DOF VEHICLE MODEL/POWERTRAIN AND BRAKES/Engine and Gear Box/Subsystem1 ==
  Engine rpm : Inport
  1-D Lookup Table : Lookup_n-D  NumberOfTableDimensions=1  BreakpointsForDimension1=Gear_numbers  Table=GR  ExtrapMethod=Clip  InternalRulePriority=Speed  RndMeth=Simplest  InputSameDT=on
  Constant : Constant  Value=initial_gear
  Constant1 : Constant  Value=enableDriverControl
  Constant2 : Constant  Value=minrpm
  Constant3 : Constant  Value=maxrpm
  Delay : Delay  DelayLength=1  InitialCondition=initial_gear
  Delay1 : Delay  DelayLength=1  InitialCondition=800
  MATLAB Function : MATLAB Function  TreatAsAtomicUnit=on
  Switch : Switch  Criteria=u2 > Threshold
  Gear No. : Outport
  Gear_Ratio : Outport  Port=2
  wires:
  Delay1/1 -> MATLAB Function/1(rpm)
  Constant2/1 -> MATLAB Function/3(minrpm)
  Delay/1 -> MATLAB Function/2(gr_no_previous)
  Constant1/1 -> Switch/2
  1-D Lookup Table/1 -> Gear_Ratio/1  "Gear_Ratio"
  MATLAB Function/1(gr_no) -> Gear No./1, Switch/1, Delay/1  "Gear No."
  Constant/1 -> Switch/3
  Switch/1 -> 1-D Lookup Table/1
  Constant3/1 -> MATLAB Function/4(maxrpm)
  Engine rpm/1 -> Delay1/1

== system VDSE_2018a/14-DOF VEHICLE MODEL/SUSPENSION/FRONT SUSPENSION/SUSPENSION FL ==
  z [m] : Inport
  Vz [m/s] : Inport  Port=2
  phi [rad] : Inport  Port=3
  phi_dot [rad/s] : Inport  Port=4
  theta [rad] : Inport  Port=5
  theta_dot [rad/s] : Inport  Port=6
  zFR [m] : Inport  Port=7
  yFL_road [m] : Inport  Port=8
  FL : Subsystem
  TIRE VERTICAL DEFLECTION : Subsystem
  fFLz [N] : Outport
  zFL_dot [m/s] : Outport  Port=2
  zFL [m] : Outport  Port=3
  wires:
  FL/2(zFL_dot [m/s]) -> TIRE VERTICAL DEFLECTION/2(zFL_dot [m/s]), zFL_dot [m/s]/1
  z [m]/1 -> FL/1(z [m])
  TIRE VERTICAL DEFLECTION/1(fFLz [N]) -> fFLz [N]/1
  theta [rad]/1 -> FL/5(theta [rad])
  zFR [m]/1 -> FL/7(zFR [m])
  Vz [m/s]/1 -> FL/2(Vz [m/s])
  yFL_road [m]/1 -> TIRE VERTICAL DEFLECTION/3(yFL_road [m]), FL/8(yFL_road [m])
  phi_dot [rad/s]/1 -> FL/4(phi_dot [rad/s])
  FL/1(zFL [m]) -> TIRE VERTICAL DEFLECTION/1(zFL [m]), zFL [m]/1
  phi [rad]/1 -> FL/3(phi [rad])
  theta_dot [rad/s]/1 -> FL/6(theta_dot [rad/s])

== system VDSE_2018a/14-DOF VEHICLE MODEL/SUSPENSION/FRONT SUSPENSION/SUSPENSION FR ==
  z [m] : Inport
  Vz [m/s] : Inport  Port=2
  phi [rad] : Inport  Port=3
  phi_dot [rad/s] : Inport  Port=4
  theta [rad] : Inport  Port=5
  theta_dot [rad/s] : Inport  Port=6
  zFL [m] : Inport  Port=7
  yFR_road [m] : Inport  Port=8
  FR : Subsystem
  TIRE VERTICAL DEFLECTION : Subsystem
  fFRz [N] : Outport
  zFR [m] : Outport  Port=2
  zFR_dot [m/s] : Outport  Port=3
  wires:
  FR/2(zFR_dot [m/s]) -> zFR_dot [m/s]/1, TIRE VERTICAL DEFLECTION/2(zFR_dot [m/s])
  yFR_road [m]/1 -> FR/8(yFR_road [m]), TIRE VERTICAL DEFLECTION/3(yFR_road [m])
  z [m]/1 -> FR/1(z [m])
  TIRE VERTICAL DEFLECTION/1(fFRz [N]) -> fFRz [N]/1
  theta [rad]/1 -> FR/5(theta [rad])
  zFL [m]/1 -> FR/7(zFL [m])
  Vz [m/s]/1 -> FR/2(Vz [m/s])
  phi_dot [rad/s]/1 -> FR/4(phi_dot [rad/s])
  FR/1(zFR [m]) -> TIRE VERTICAL DEFLECTION/1(zFR [m]), zFR [m]/1
  phi [rad]/1 -> FR/3(phi [rad])
  theta_dot [rad/s]/1 -> FR/6(theta_dot [rad/s])

== system VDSE_2018a/14-DOF VEHICLE MODEL/SUSPENSION/Load Transfer/Coupling of load transfer and suspension reaction ==
  Longidutinal Load Transfer [N] : Inport
  Lateral Load Transfer - Front [N] : Inport  Port=2
  Lateral Load Transfer - Rear [N] : Inport  Port=3
  <fFLz [N]> : Inport  Port=4
  <fFRz [N]> : Inport  Port=5
  <fRLz [N]> : Inport  Port=6
  <fRRz [N]> : Inport  Port=7
  Add{,1..4} (5 alike) : Sum
  Add5 : Sum  Inputs=+-
  Add6 : Sum  Inputs=-+
  Add7 : Sum  Inputs=--
  Lateral Load Transfer - Front [N]1 : InportShadow  Port=2
  Lateral Load Transfer - Rear [N]1 : InportShadow  Port=3
  Longidutinal Load Transfer [N]1 : InportShadow
  Longidutinal Load Transfer [N]2 : InportShadow
  Longidutinal Load Transfer [N]3 : InportShadow
  FLz_Overall [N] : Outport
  FRz_Overall [N] : Outport  Port=2
  RLz_Overall [N] : Outport  Port=3
  RRz_Overall [N] : Outport  Port=4
  wires:
  <fFRz [N]>/1 -> Add1/2
  Lateral Load Transfer - Rear [N]/1 -> Add5/2
  Longidutinal Load Transfer [N]/1 -> Add7/1
  Add7/1 -> Add/1  "FL Dynamic LT"
  Lateral Load Transfer - Front [N]/1 -> Add7/2
  Add4/1 -> Add3/1  "RR Dynamic LT"
  Add6/1 -> Add1/1  "FR Dynamic LT"
  Add5/1 -> Add2/1  "RL Dynamic LT"
  <fRRz [N]>/1 -> Add3/2
  <fFLz [N]>/1 -> Add/2
  <fRLz [N]>/1 -> Add2/2
  Add1/1 -> FRz_Overall [N]/1  "FRz_Overall [N]"
  Add3/1 -> RRz_Overall [N]/1  "RRz_Overall [N]"
  Add/1 -> FLz_Overall [N]/1  "FLz_Overall [N]"
  Add2/1 -> RLz_Overall [N]/1  "RLz_Overall [N]"
  Longidutinal Load Transfer [N]1/1 -> Add6/1
  Longidutinal Load Transfer [N]2/1 -> Add5/1
  Longidutinal Load Transfer [N]3/1 -> Add4/1
  Lateral Load Transfer - Front [N]1/1 -> Add6/2
  Lateral Load Transfer - Rear [N]1/1 -> Add4/2

== system VDSE_2018a/14-DOF VEHICLE MODEL/SUSPENSION/Load Transfer/Dynamic Lateral Load Transfer - Front ==
  ay [m/s^2] : Inport
  Add : Sum
  Gain : Gain  Gain=lR/(lR+lF)
  Gain1 : Gain  Gain=2*mF*huFcog/wF
  Gain2 : Gain  Gain=m*hrcF/wF
  Lat. Dynamic Transfer [N] : Outport
  wires:
  ay [m/s^2]/1 -> Gain2/1, Gain1/1
  Gain2/1 -> Gain/1
  Add/1 -> Lat. Dynamic Transfer [N]/1
  Gain1/1 -> Add/2
  Gain/1 -> Add/1

== system VDSE_2018a/14-DOF VEHICLE MODEL/SUSPENSION/Load Transfer/Dynamic Lateral Load Transfer - Rear ==
  ay [m/s^2] : Inport
  Add : Sum
  Gain : Gain  Gain=lF/(lR+lF)
  Gain1 : Gain  Gain=2*mR*huRcog/wR
  Gain2 : Gain  Gain=m*hrcR/wR
  Lat. Dynamic Transfer [N] : Outport
  wires:
  Add/1 -> Lat. Dynamic Transfer [N]/1
  Gain1/1 -> Add/2
  ay [m/s^2]/1 -> Gain2/1, Gain1/1
  Gain2/1 -> Gain/1
  Gain/1 -> Add/1

== system VDSE_2018a/14-DOF VEHICLE MODEL/SUSPENSION/Load Transfer/Dynamic Longitudinal Load Transfer ==
  ax [m/s^2] : Inport
  Add : Sum
  Gain : Gain  Gain=1/2*hpc*m/(lF+lR)/2
  Gain1 : Gain  Gain=(mF*huFcog + mR*huRcog)/(lF+lR)
  Long. Dynamic Transfer [N] : Outport
  wires:
  ax [m/s^2]/1 -> Gain1/1, Gain/1
  Gain/1 -> Add/1
  Add/1 -> Long. Dynamic Transfer [N]/1
  Gain1/1 -> Add/2

== system VDSE_2018a/14-DOF VEHICLE MODEL/SUSPENSION/REAR SUSPENSION/SUSPENSION RL ==
  z [m] : Inport
  Vz [m/s] : Inport  Port=2
  phi [rad] : Inport  Port=3
  phi_dot [rad/s] : Inport  Port=4
  theta [rad] : Inport  Port=5
  theta_dot [rad/s] : Inport  Port=6
  zRR [m] : Inport  Port=7
  yRL_road [m] : Inport  Port=8
  RL : Subsystem
  TIRE VERTICAL DEFLECTION : Subsystem
  fRLz [N] : Outport
  zRL_dot [m/s] : Outport  Port=2
  zRL [m] : Outport  Port=3
  wires:
  RL/2(zRL_dot [m/s]) -> TIRE VERTICAL DEFLECTION/2(zRL_dot [m/s]), zRL_dot [m/s]/1
  z [m]/1 -> RL/1(z [m])
  TIRE VERTICAL DEFLECTION/1(fRLz [N]) -> fRLz [N]/1  "fRLz [N]"
  theta [rad]/1 -> RL/5(theta [rad])
  zRR [m]/1 -> RL/7(zRR [m])
  Vz [m/s]/1 -> RL/2(Vz [m/s])
  yRL_road [m]/1 -> TIRE VERTICAL DEFLECTION/3(yRL_road [m]), RL/8(yRL_road [m])
  phi_dot [rad/s]/1 -> RL/4(phi_dot [rad/s])
  RL/1(zRL [m]) -> TIRE VERTICAL DEFLECTION/1(zRL [m]), zRL [m]/1
  phi [rad]/1 -> RL/3(phi [rad])
  theta_dot [rad/s]/1 -> RL/6(theta_dot [rad/s])

== system VDSE_2018a/14-DOF VEHICLE MODEL/SUSPENSION/REAR SUSPENSION/SUSPENSION RR ==
  z [m] : Inport
  Vz [m/s] : Inport  Port=2
  phi [rad] : Inport  Port=3
  phi_dot [rad/s] : Inport  Port=4
  theta [rad] : Inport  Port=5
  theta_dot [rad/s] : Inport  Port=6
  zRL [m] : Inport  Port=7
  yRR_road [m] : Inport  Port=8
  RR : Subsystem
  TIRE VERTICAL DEFLECTION : Subsystem
  fRRz [N] : Outport
  zRR [m] : Outport  Port=2
  zRR_dot [m/s] : Outport  Port=3
  wires:
  RR/2(zRR_dot [m/s]) -> TIRE VERTICAL DEFLECTION/2(zRR_dot [m/s]), zRR_dot [m/s]/1
  yRR_road [m]/1 -> TIRE VERTICAL DEFLECTION/3(yRR_road [m]), RR/8(yRR_road [m])
  z [m]/1 -> RR/1(z [m])
  TIRE VERTICAL DEFLECTION/1(fRRz [N]) -> fRRz [N]/1
  theta [rad]/1 -> RR/5(theta [rad])
  zRL [m]/1 -> RR/7(zRL [m])
  Vz [m/s]/1 -> RR/2(Vz [m/s])
  phi_dot [rad/s]/1 -> RR/4(phi_dot [rad/s])
  RR/1(zRR [m]) -> TIRE VERTICAL DEFLECTION/1(zRR [m]), zRR [m]/1
  phi [rad]/1 -> RR/3(phi [rad])
  theta_dot [rad/s]/1 -> RR/6(theta_dot [rad/s])

== system VDSE_2018a/14-DOF VEHICLE MODEL/WHEEL ASSEMBLY/WHEEL ASSEMBLY BCD/SIDE SLIP ANGLE CALCULATION ==
  Vx [m/s] : Inport
  Vy [m/s] : Inport  Port=2
  Add : Sum
  Atan2 : Trigonometry  Operator=atan2
  Clock : Clock
  Constant : Constant  Value=enableLongDynamics
  Constant1 : Constant  Value=Vx0
  Constant2 : Constant  Value=0
  Sqrt : Sqrt  SaturateOnIntegerOverflow=on
  Square : Math  Operator=square  SaturateOnIntegerOverflow=on
  Square1 : Math  Operator=square  SaturateOnIntegerOverflow=on
  Switch : Switch  Criteria=u2 > Threshold
  Switch1 : Switch  Criteria=u2 > Threshold  Threshold=0.01
  Vy [m/s]1 : InportShadow  Port=2
  V [m/s] : Outport
  beta [rad] : Outport  Port=2
  wires:
  Clock/1 -> Switch1/2
  Constant2/1 -> Switch1/3
  Switch1/1 -> Switch/2
  Constant1/1 -> Switch/3
  Constant/1 -> Switch1/1
  Switch/1 -> Atan2/2, Square/1
  Square1/1 -> Add/2
  Square/1 -> Add/1
  Vy [m/s]/1 -> Square1/1
  Vx [m/s]/1 -> Switch/1
  Add/1 -> Sqrt/1
  Sqrt/1 -> V [m/s]/1
  Atan2/1 -> beta [rad]/1
  Vy [m/s]1/1 -> Atan2/1

== system VDSE_2018a/14-DOF VEHICLE MODEL/WHEEL ASSEMBLY/WHEEL ASSEMBLY BCD/TIRE PARAMETERS ==
  Constant : Constant  Value=Bxf
  Constant1 : Constant  Value=Cxf
  Constant10 : Constant  Value=Cyr
  Constant11 : Constant  Value=Dyr
  Constant2 : Constant  Value=Dxf
  Constant3 : Constant  Value=Bxr
  Constant4 : Constant  Value=Cxr
  Constant5 : Constant  Value=Dxr
  Constant6 : Constant  Value=Byf
  Constant7 : Constant  Value=Cyf
  Constant8 : Constant  Value=Dyf
  Constant9 : Constant  Value=Byr
  Bxf : Outport
  Cxf : Outport  Port=2
  Dxf : Outport  Port=3
  Bxr : Outport  Port=4
  Cxr : Outport  Port=5
  Dxr : Outport  Port=6
  Byf : Outport  Port=7
  Cyf : Outport  Port=8
  Dyf : Outport  Port=9
  Byr : Outport  Port=10
  Cyr : Outport  Port=11
  Dyr : Outport  Port=12
  wires:
  Constant/1 -> Bxf/1
  Constant1/1 -> Cxf/1
  Constant2/1 -> Dxf/1
  Constant5/1 -> Dxr/1
  Constant4/1 -> Cxr/1
  Constant3/1 -> Bxr/1
  Constant9/1 -> Byr/1
  Constant10/1 -> Cyr/1
  Constant11/1 -> Dyr/1
  Constant8/1 -> Dyf/1
  Constant7/1 -> Cyf/1
  Constant6/1 -> Byf/1

== system VDSE_2018a/14-DOF VEHICLE MODEL/WHEEL ASSEMBLY/WHEEL ASSEMBLY MFEVAL/SIDE SLIP ANGLE CALCULATION ==
  Vx [m/s] : Inport
  Vy [m/s] : Inport  Port=2
  Add : Sum
  Atan2 : Trigonometry  Operator=atan2
  Clock : Clock
  Constant : Constant  Value=enableLongDynamics
  Constant1 : Constant  Value=Vx0
  Constant2 : Constant  Value=0
  Sqrt : Sqrt  SaturateOnIntegerOverflow=on
  Square : Math  Operator=square  SaturateOnIntegerOverflow=on
  Square1 : Math  Operator=square  SaturateOnIntegerOverflow=on
  Switch : Switch  Criteria=u2 > Threshold
  Switch1 : Switch  Criteria=u2 > Threshold  Threshold=0.01
  Vy [m/s]1 : InportShadow  Port=2
  V [m/s] : Outport
  beta [rad] : Outport  Port=2
  wires:
  Clock/1 -> Switch1/2
  Constant2/1 -> Switch1/3
  Switch1/1 -> Switch/2
  Constant1/1 -> Switch/3
  Constant/1 -> Switch1/1
  Square1/1 -> Add/2
  Square/1 -> Add/1
  Vy [m/s]/1 -> Square1/1
  Vx [m/s]/1 -> Switch/1
  Add/1 -> Sqrt/1
  Atan2/1 -> beta [rad]/1
  Vy [m/s]1/1 -> Atan2/1
  Switch/1 -> Atan2/2, Square/1
  Sqrt/1 -> V [m/s]/1

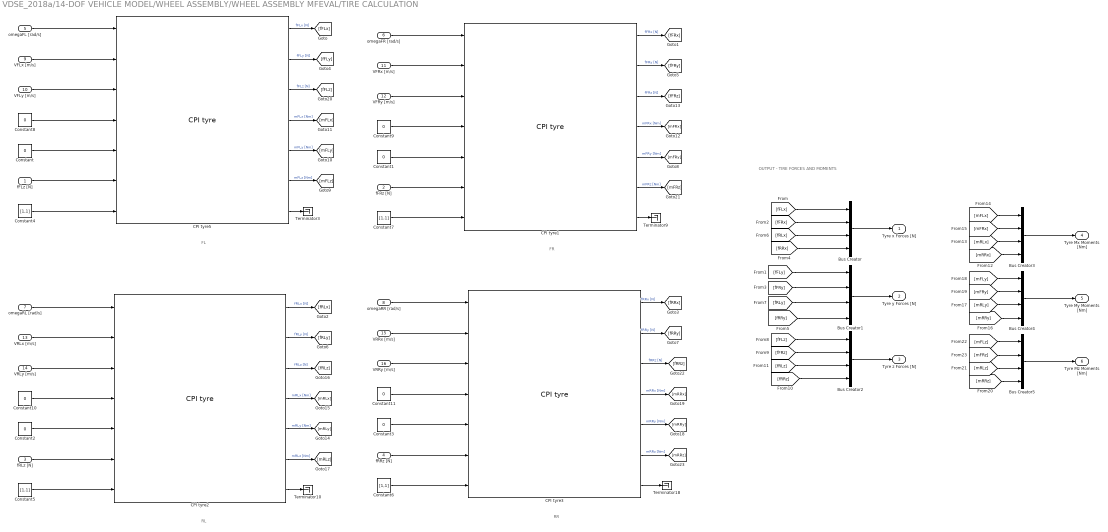
== system VDSE_2018a/14-DOF VEHICLE MODEL/WHEEL ASSEMBLY/WHEEL ASSEMBLY MFEVAL/TIRE CALCULATION ==
  note: RR
  note: RL
  note: FR
  note: FL
  note: OUTPUT - TIRE FORCES AND MOMENTS
  fFLz [N] : Inport
  fFRz [N] : Inport  Port=2
  fRLz [N] : Inport  Port=3
  fRRz [N] : Inport  Port=4
  omegaFL [rad/s] : Inport  Port=5
  omegaFR [rad/s] : Inport  Port=6
  omegaRL [rad/s] : Inport  Port=7
  omegaRR [rad/s] : Inport  Port=8
  VFLx [m/s] : Inport  Port=9
  VFLy [m/s] : Inport  Port=10
  VFRx [m/s] : Inport  Port=11
  VFRy [m/s] : Inport  Port=12
  VRLx [m/s] : Inport  Port=13
  VRLy [m/s] : Inport  Port=14
  VRRx [m/s] : Inport  Port=15
  VRRy [m/s] : Inport  Port=16
  Bus Creator{,1..5} (6 alike) : BusCreator  Inputs=4
  CPI tyre1 : mfeval_LIB/CPI tyre  Description=Magic Formula 6.1.2 tyre model including relaxation length and transient calculations  userParameterSource=tir_file_front  userSide=2 right  userDynamics=1 steady state  userUseMode=1 combined  enablePressure=off  userPressure=2.3
      settings: SourceProductName=MFeval Library
  CPI tyre2 : mfeval_LIB/CPI tyre  Description=Magic Formula 6.1.2 tyre model including relaxation length and transient calculations  userParameterSource=tir_file_rear  userSide=1 left  userDynamics=1 steady state  userUseMode=1 combined  enablePressure=off  userPressure=2.3
      settings: SourceProductName=MFeval Library
  CPI tyre3 : mfeval_LIB/CPI tyre  Description=Magic Formula 6.1.2 tyre model including relaxation length and transient calculations  userParameterSource=tir_file_rear  userSide=2 right  userDynamics=1 steady state  userUseMode=1 combined  enablePressure=off  userPressure=2.3
      settings: SourceProductName=MFeval Library
  CPI tyre5 : mfeval_LIB/CPI tyre  Description=Magic Formula 6.1.2 tyre model including relaxation length and transient calculations  userParameterSource=tir_file_front  userSide=1 left  userDynamics=1 steady state  userUseMode=1 combined  enablePressure=off  userPressure=2.3
      settings: SourceProductName=MFeval Library
  Constant{,1..3,8..11} (8 alike) : Constant  Value=0
  Constant{4..7} (4 alike) : Constant  Value=[1,1]
  Terminator{3,9..10,18} (4 alike) : Terminator
  Tyre x Forces [N] : Outport
  Tyre y Forces [N] : Outport  Port=2
  Tyre z Forces [N] : Outport  Port=3
  Tyre Mx Moments [Nm] : Outport  Port=4
  Tyre My Moments [Nm] : Outport  Port=5
  Tyre Mz Moments [Nm] : Outport  Port=6
  wires:
  Constant11/1 -> CPI tyre3/4
  Constant10/1 -> CPI tyre2/4
  Constant9/1 -> CPI tyre1/4
  Constant8/1 -> CPI tyre5/4
  CPI tyre3/3 -> [fRRz]  "fRRz [N]"
  CPI tyre3/6 -> [mRRz]  "mRRz [Nm]"
  CPI tyre3/4 -> [mRRx]  "mRRx [Nm]"
  CPI tyre3/5 -> [mRRy]  "mRRy [Nm]"
  CPI tyre2/3 -> [fRLz]  "fRLz [N]"
  CPI tyre2/6 -> [mRLz]  "mRLz [Nm]"
  CPI tyre2/4 -> [mRLx]  "mRLx [Nm]"
  CPI tyre2/5 -> [mRLy]  "mRLy [Nm]"
  CPI tyre1/3 -> [fFRz]  "fFRz [N]"
  CPI tyre1/6 -> [mFRz]  "mFRz [Nm]"
  CPI tyre1/4 -> [mFRx]  "mFRx [Nm]"
  CPI tyre1/5 -> [mFRy]  "mFRy [Nm]"
  CPI tyre5/3 -> [fFLz]  "fFLz [N]"
  CPI tyre5/4 -> [mFLx]  "mFLx [Nm]"
  CPI tyre5/5 -> [mFLy]  "mFLy [Nm]"
  Bus Creator5/1 -> Tyre Mz Moments [Nm]/1
  [mFRz] -> Bus Creator5/2
  [mRLz] -> Bus Creator5/3
  [mRRz] -> Bus Creator5/4
  [mFLz] -> Bus Creator5/1
  [mFLy] -> Bus Creator4/1
  [mRRy] -> Bus Creator4/4
  [mRLy] -> Bus Creator4/3
  [mFRy] -> Bus Creator4/2
  Bus Creator4/1 -> Tyre My Moments [Nm]/1
  Bus Creator3/1 -> Tyre Mx Moments [Nm]/1
  [mFRx] -> Bus Creator3/2
  [mRLx] -> Bus Creator3/3
  [mRRx] -> Bus Creator3/4
  [mFLx] -> Bus Creator3/1
  [fFLz] -> Bus Creator2/1
  [fRRz] -> Bus Creator2/4
  [fRLz] -> Bus Creator2/3
  [fFRz] -> Bus Creator2/2
  Bus Creator2/1 -> Tyre z Forces [N]/1
  Bus Creator1/1 -> Tyre y Forces [N]/1
  Bus Creator/1 -> Tyre x Forces [N]/1
  [fFRy] -> Bus Creator1/2
  [fRLy] -> Bus Creator1/3
  [fRRy] -> Bus Creator1/4
  [fFLy] -> Bus Creator1/1
  [fRRx] -> Bus Creator/4
  [fRLx] -> Bus Creator/3
  [fFRx] -> Bus Creator/2
  [fFLx] -> Bus Creator/1
  CPI tyre3/2 -> [fRRy]  "fRRy [N]"
  CPI tyre2/2 -> [fRLy]  "fRLy [N]"
  CPI tyre1/2 -> [fFRy]  "fFRy [N]"
  CPI tyre5/2 -> [fFLy]  "fFLy [N]"
  CPI tyre2/1 -> [fRLx]  "fRLx [N]"
  CPI tyre3/1 -> [fRRx]  "fRRx [N]"
  CPI tyre1/1 -> [fFRx]  "fFRx [N]"
  CPI tyre5/1 -> [fFLx]  "fFLx [N]"
  CPI tyre3/7 -> Terminator18/1
  CPI tyre2/7 -> Terminator10/1
  CPI tyre1/7 -> Terminator9/1
  CPI tyre5/7 -> Terminator3/1
  CPI tyre5/6 -> [mFLz]  "mFLz [Nm]"
  VRRx [m/s]/1 -> CPI tyre3/2
  VRRy [m/s]/1 -> CPI tyre3/3
  VRLy [m/s]/1 -> CPI tyre2/3
  VRLx [m/s]/1 -> CPI tyre2/2
  VFRy [m/s]/1 -> CPI tyre1/3
  VFRx [m/s]/1 -> CPI tyre1/2
  VFLx [m/s]/1 -> CPI tyre5/2
  VFLy [m/s]/1 -> CPI tyre5/3
  omegaRR [rad/s]/1 -> CPI tyre3/1
  omegaRL [rad/s]/1 -> CPI tyre2/1
  omegaFR [rad/s]/1 -> CPI tyre1/1
  omegaFL [rad/s]/1 -> CPI tyre5/1
  Constant7/1 -> CPI tyre1/7
  Constant6/1 -> CPI tyre3/7
  Constant5/1 -> CPI tyre2/7
  Constant4/1 -> CPI tyre5/7
  Constant3/1 -> CPI tyre3/5
  Constant2/1 -> CPI tyre2/5
  Constant1/1 -> CPI tyre1/5
  Constant/1 -> CPI tyre5/5
  fFLz [N]/1 -> CPI tyre5/6
  fRLz [N]/1 -> CPI tyre2/6
  fRRz [N]/1 -> CPI tyre3/6
  fFRz [N]/1 -> CPI tyre1/6

== system VDSE_2018a/14-DOF VEHICLE MODEL/WHEEL ASSEMBLY/WHEEL ASSEMBLY PACEIJKA/SIDE SLIP ANGLE CALCULATION ==
  Vx [m/s] : Inport
  Vy [m/s] : Inport  Port=2
  Add : Sum
  Atan2 : Trigonometry  Operator=atan2
  Clock : Clock
  Constant : Constant  Value=enableLongDynamics
  Constant1 : Constant  Value=Vx0
  Constant2 : Constant  Value=0
  Sqrt : Sqrt  SaturateOnIntegerOverflow=on
  Square : Math  Operator=square  SaturateOnIntegerOverflow=on
  Square1 : Math  Operator=square  SaturateOnIntegerOverflow=on
  Switch : Switch  Criteria=u2 > Threshold
  Switch1 : Switch  Criteria=u2 > Threshold  Threshold=0.01
  Vy [m/s]1 : InportShadow  Port=2
  V [m/s] : Outport
  beta [rad] : Outport  Port=2
  wires:
  Vy [m/s]1/1 -> Atan2/1
  Atan2/1 -> beta [rad]/1
  Sqrt/1 -> V [m/s]/1
  Add/1 -> Sqrt/1
  Vx [m/s]/1 -> Switch/1
  Vy [m/s]/1 -> Square1/1
  Square/1 -> Add/1
  Square1/1 -> Add/2
  Switch/1 -> Atan2/2, Square/1
  Constant/1 -> Switch1/1
  Constant1/1 -> Switch/3
  Switch1/1 -> Switch/2
  Constant2/1 -> Switch1/3
  Clock/1 -> Switch1/2
